simulink model "actuator_level_gripper"  (R2016a)
settings: Solver=FixedStepDiscrete  SolverMode=SingleTasking  StartTime=0.0  StopTime=inf  RelTol=1e-3
settings Model: SimulationMode=external  ExtModeTrigDuration=2  Creator=Joshua  LastModifiedBy=dell
settings DataIOCC: LimitDataPoints=on  SaveFormat=Array
settings OptimizationCC: OptimizeModelRefInitCode=on  LifeSpan=Inf  MaxStackSize=64
settings DebuggingCC: UnderspecifiedInitializationDetection=Classic  MergeDetectMultiDrivingBlocksExec=none
settings HardwareCC: ProdBitPerInt=16  ProdBitPerPointer=16  ProdLargestAtomicFloat=None  ProdWordSize=8  ProdHWDeviceType=Atmel->AVR
settings ModelReferenceCC: PropagateSignalLabelsOutOfModel=off
settings RTWCC: SystemTargetFile=ert.tlc  HardwareBoard=Arduino Mega 2560  TemplateMakefile=ert_default_tmf  GenerateReport=on  RTWVerbose=off  Toolchain=Arduino AVR v1.6.1  BuildConfiguration=Faster Runs  IncludeHyperlinkInReport=on  LaunchReport=on  GenerateTraceInfo=on  GenerateTraceReport=on  GenerateTraceReportSl=on  GenerateTraceReportSf=on  GenerateTraceReportEml=on
settings CodeAppCC: ForceParamTrailComments=on  IgnoreCustomStorageClasses=off  OperatorAnnotations=on  SimulinkDataObjDesc=on  SFDataObjDesc=on  MATLABFcnDesc=on  InsertBlockDesc=on  MATLABSourceComments=on
settings ERTTargetCC: SupportContinuousTime=on  SupportVariableSizeSignals=on
settings ConfigComp: CovModelRefEnable=Off

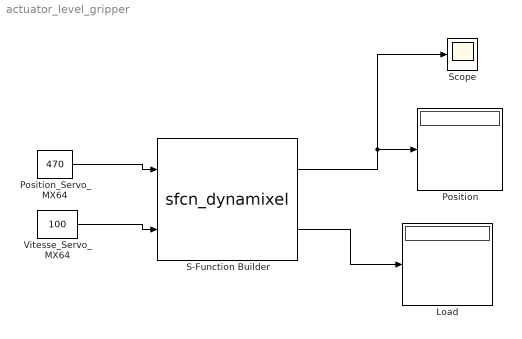
== system actuator_level_gripper ==
  Load : Display
  Position : Display
  Position_Servo_MX64 : Constant  Value=470  OutDataTypeStr=int16
  S-Function Builder : S-Function  InitFcn=try, set_param(gcb,'FunctionName','sfcn_dynamixel'), end  FunctionName=sfcn_dynamixel  Parameters=int8(2),uint32(1000000),int8([1 ]),uint32(200)  SFunctionModules=sfcn_dynamixel_wrapper  SFunctionDeploymentMode=off  EnableBusSupport=off  mask(Dynamixel driver){portNumber=Serial Port 2, baudrate=1000000, tx=200, identity=[1 2 3 4]}
      mask prompts: portNumber "Serial Port Number (Arduino Mega 2560):"; baudrate "Baud Rate:"; tx "TX Delay Time:"; identity "ID*:"
      mask help:
      | This block provides a driver to control robots built by Dynamixel servos, with a discrete sample time of 0.05 seconds.
      | The first input "q" represents the desired position.
      | The output shows a column vector with the joint angle of each servo in real time.
      mask init:
      | val = [[.9  0.75 0.75 1 1 .9 .9 1]',[1 1 0.75 0.75 .9 .9 1 .9]'];try , sys = get_param(gcb,'SfunBuilderFcnName');if isempty(sys), sys = get_param(gcb,'FunctionName'); end,catch, sys = get_param(gcb,'FunctionName'); end
      settings: CopyFcn=set_param(gcbh,'LinkStatus','none')  PreSaveFcn=try, set_param(gcb,'FunctionName','sfcn_dynamixel'), end  OpenFcn=sfunctionwizard(gcbh)
      mask TypeOptions portNumber: Serial Port 1 | Serial Port 2 | Serial Port 3
      mask Display: plot(val(:,1),val(:,2)),disp(sys), port_label('input',1,'qd'), port_label('input',2,'dqd'), port_label('output',1,'q'), port_label('output',2,'load')
  Scope : Scope
  Vitesse_Servo_MX64 : Constant  Value=100  OutDataTypeStr=int16
  wires:
  S-Function Builder/1 -> Scope/1, Position/1
  Vitesse_Servo_MX64/1 -> S-Function Builder/2
  S-Function Builder/2 -> Load/1
  Position_Servo_MX64/1 -> S-Function Builder/1
